simulink model "SingleTrackCANoe"  (R2021b)
settings: Solver=ode1  StartTime=0  StopTime=2  FixedStep=1.0000000000000000e-003  RelTol=1e-3
InitFcn:
  | sampleTime = str2double(get_param(bdroot, 'FixedStep'));
undefined symbols (not defined in the file or in its folder): AccPedalPos, BrakePedalPos, BrakeSwitch, DiscIntNeverNeededParam, DYNA4, EngSpd, IgnitionSwitch, InitialGear, InitialSpeed, IntendedEngTrq, LeftIndicator, MainBrakePress, MaxGear, MDL, MinGear, RefAcc, RefLane, RefLatPos, RefPath, RefPathCurv, RefSpd, RefSpdPreview, RefSpdRetrospect, RightIndicator, SteeringWheelAng, SteeringWheelTrq, UserDefinedRefValue, vm_const
libraries: UtilitiesLibrary x62, simulink x18, WheelSystemModules x14, LongitudinalControllerModules x13, LateralControllerModules x7, AnimationBusselectorModules x5, EnvironmentModules x5, BasicEngineControlModules x5, MiscellaneousControlModules x5, Animation3Modules x4, AuxiliariesModules x4, ReducedTireModules x4
(part 13 of 34)

== system SingleTrackCANoe/SimulationModel/Vehicle/Engine/EnginePhysics ==
  fromEngineControlUnit : Inport
  fromCTRL : Inport  Port=2
  fromEnvironment : Inport  Port=3
  fromChassis : Inport  Port=4
  fromDrivetrain : Inport  Port=5
  fromElectricalSystem : Inport  Port=6
  ConsumptionCalculation : EngineLookupTableModules/ConsumptionCalculation  FuelConsumptionLimStandEu=50  FuelConsumptionLimitCutoffUS=50
  DynaComponentInfo : Subsystem  Tag=DynaComponentInfo
      mask init:
      | data= get_param(gcb, 'UserData');
      settings: OpenFcn=DYNA4.ModelHandling.Component.ShowEditComponentInformationDialog(gcb);
      mask Display: disp(['Type = ', data.type, '\nGroup = ', data.group, '\nName = ', data.name ])
  EnginePhysicsOutput : Subsystem  Tag=TESIS DYNAware Interface Block  mask{NeedsUpdate=off, SignalInfo=|}
      mask SignalInfo=|
      | {
      |   "Version": "4.6",
      |   "MuxedOutputBusName": "EnginePhysics",
      |   "MuxedInputBusName": "input",
      |   "MuxedInputSelected": false,
      |   "MuxedOutputSelected": true,
      |   "SignalData": [
      |     {
      |       "initialValue": "0.0",
      |       "name": "Mechanics",
      |       "comment": "",
      |       "minString": "",
      |       "maxString": "",
      |       "width": -1,
      |       "dataType": 0,
      |       "signalType": 1,
      |       "createSignal": false,
      |       "outputName": "Mechanics",
      |       "generateSignalAccessBlock": false,
      |       "accessId": "$(parentId).$(blockName).$(outputName)"
      |     },
      |     {
      |       "initialValue": "0.0",
      |       "name": "ValidityStatus",
      |       "comment": "",
      |       "minString": "",
      |       "maxString": "",
      |       "width": -1,
      |       "dataType": 0,
      |       "signalType": 1,
      |       "createSignal": false,
      |       "outputName": "ValidityStatus",
      |       "generateSignalAccessBlock": false,
      |       "accessId": "$(parentId).$(blockName).$(outputName)"
      |     },
      |     {
      |       "initialValue": "0.0",
      |       "name": "FuelSystem",
      |       "comment": "",
      |       "minString": "",
      |       "maxString": "",
      |       "width": -1,
      |       "dataType": 0,
      |       "signalType": 1,
      |       "createSignal": false,
      |       "outputName": "FuelSystem",
      |       "generateSignalAccessBlock": false,
      |       "accessId": "$(parentId).$(blockName).$(outputName)"
      |     }
      |   ]
      | }
      mask prompts: NeedsUpdate "Specify, if subsystem content needs to be updated"; SignalInfo "Signal Info (json)"
      mask help: DYNA4 Interface Block Version 4.6
      mask init:
      | blockName = get_param(gcbh, 'Name');
      | parentId = DYNA4.ModelHandling.AccessID.getFromHierarchy(gcbh);
      | TD.InterfaceBlock.ModelCallbacks.GenerateContent(gcb);
      settings: DeleteFcn=TD.InterfaceBlock.ModelCallbacks.CloseGUI( gcbh );  NameChangeFcn=TD.InterfaceBlock.ModelCallbacks.BlockRenamedHandler(gcbh);  OpenFcn=TD.InterfaceBlock.ModelCallbacks.OpenGUI( gcbh );  CloseFcn=TD.InterfaceBlock.ModelCallbacks.CloseGUI( gcbh );
      mask Display:
      | image('InterfaceBlock.png','center');
      | port_label('input',1, 'Mechanics');
      | port_label('input',2, 'ValidityStatus');
      | port_label('input',3, 'FuelSystem');
      | port_label('output',1, 'EnginePhysics');
  FuelSystemOutput : Subsystem  Tag=TESIS DYNAware Interface Block  mask{NeedsUpdate=off, SignalInfo=|}
      mask SignalInfo=|
      | {
      |   "Version": "4.6",
      |   "MuxedOutputBusName": "FuelSystem",
      |   "MuxedInputBusName": "input",
      |   "MuxedInputSelected": false,
      |   "MuxedOutputSelected": true,
      |   "SignalData": [
      |     {
      |       "initialValue": "0.0",
      |       "name": "FuelMassFlow[kg/s]",
      |       "comment": "",
      |       "minString": "",
      |       "maxString": "",
      |       "width": 1,
      |       "dataType": 0,
      |       "signalType": 0,
      |       "createSignal": false,
      |       "outputName": "FuelMassFlow[kg/s]",
      |       "generateSignalAccessBlock": false,
      |       "accessId": "$(parentId).$(blockName).$(outputName)"
      |     },
      |     {
      |       "initialValue": "0.0",
      |       "name": "FuelMass[kg]",
      |       "comment": "",
      |       "minString": "",
      |       "maxString": "",
      |       "width": 1,
      |       "dataType": 0,
      |       "signalType": 0,
      |       "createSignal": false,
      |       "outputName": "FuelMass[kg]",
      |       "generateSignalAccessBlock": false,
      |       "accessId": "$(parentId).$(blockName).$(outputName)"
      |     },
      |     {
      |       "initialValue": "0.0",
      |       "name": "CurrFuelConsumEu[l/100km]",
      |       "comment": "",
      |       "minString": "",
      |       "maxString": "",
      |       "width": 1,
      |       "dataType": 0,
      |       "signalType": 0,
      |       "createSignal": false,
      |       "outputName": "CurrFuelConsumEu[l/100km]",
      |       "generateSignalAccessBlock": false,
      |       "accessId": "$(parentId).$(blockName).$(outputName)"
      |     },
      |     {
      |       "initialValue": "0.0",
      |       "name": "CurrFuelConsumUs[mpg]",
      |       "comment": "",
      |       "minString": "",
      |       "maxString": "",
      |       "width": 1,
      |       "dataType": 0,
      |       "signalType": 0,
      |       "createSignal": false,
      |       "outputName": "CurrFuelConsumUs[mpg]",
      |       "generateSignalAccessBlock": false,
      |       "accessId": "$(parentId).$(blockName).$(outputName)"
      |     },
      |     {
      |       "initialValue": "0.0",
      |       "name": "AvgFuelConsumEu[l/100km]",
      |       "comment": "",
      |       "minString": "",
      |       "maxString": "",
      |       "width": 1,
      |       "dataType": 0,
      |       "signalType": 0,
      |       "createSignal": false,
      |       "outputName": "AvgFuelConsumEu[l/100km]",
      |       "generateSignalAccessBlock": false,
      |       "accessId": "$(parentId).$(blockName).$(outputName)"
      |     },
      |     {
      |       "initialValue": "0.0",
      |       "name": "AvgFuelConsumUs[mpg]",
      |       "comment": "",
      |       "minString": "",
      |       "maxString": "",
      |       "width": 1,
      |       "dataType": 0,
      |       "signalType": 0,
      |       "createSignal": false,
      |       "outputName": "AvgFuelConsumUs[mpg]",
      |       "generateSignalAccessBlock": false,
      |       "accessId": "$(parentId).$(blockName).$(outputName)"
      |     },
      |     {
      |       "initialValue": "0.0",
      |       "name": "Efficiency[-]",
      |       "comment": "",
      |       "minString": "",
      |       "maxString": "",
      |       "width": 1,
      |       "dataType": 0,
      |       "signalType": 0,
      |       "createSignal": false,
      |       "outputName": "Efficiency[-]",
      |       "generateSignalAccessBlock": false,
      |       "accessId": "$(parentId).$(blockName).$(outputName)"
      |     },
      |     {
      |       "initialValue": "0.0",
      |       "name": "FuelDensity[kg/m**3]",
      |       "comment": "",
      |       "minString": "",
      |       "maxString": "",
      |       "width": 1,
      |       "dataType": 0,
      |       "signalType": 0,
      |       "createSignal": false,
      |       "outputName": "FuelDensity[kg/m**3]",
      |       "generateSignalAccessBlock": false,
      |       "accessId": "$(parentId).$(blockName).$(outputName)"
      |     }
      |   ]
      | }
      mask prompts: NeedsUpdate "Specify, if subsystem content needs to be updated"; SignalInfo "Signal Info (json)"
      mask help: DYNA4 Interface Block Version 4.6
      mask init:
      | blockName = get_param(gcbh, 'Name');
      | parentId = DYNA4.ModelHandling.AccessID.getFromHierarchy(gcbh);
      | TD.InterfaceBlock.ModelCallbacks.GenerateContent(gcb);
      settings: DeleteFcn=TD.InterfaceBlock.ModelCallbacks.CloseGUI( gcbh );  NameChangeFcn=TD.InterfaceBlock.ModelCallbacks.BlockRenamedHandler(gcbh);  OpenFcn=TD.InterfaceBlock.ModelCallbacks.OpenGUI( gcbh );  CloseFcn=TD.InterfaceBlock.ModelCallbacks.CloseGUI( gcbh );
      mask Display:
      | image('InterfaceBlock.png','center');
      | port_label('input',1, 'FuelMassFlow[kg/s]');
      | port_label('input',2, 'FuelMass[kg]');
      | port_label('input',3, 'CurrFuelConsumEu[l/100km]');
      | port_label('input',4, 'CurrFuelConsumUs[mpg]');
      | port_label('input',5, 'AvgFuelConsumEu[l/100km]');
      | port_label('input',6, 'AvgFuelConsumUs[mpg]');
      | port_label('input',7, 'Efficiency[-]');
      | port_label('input',8, 'FuelDensity[kg/m**3]');
      | port_label('output',1, 'FuelSystem');
  InputFromChassis : Subsystem  Tag=TESIS DYNAware Interface Block  mask{NeedsUpdate=off, SignalInfo=|}
      mask SignalInfo=|
      | {
      |   "Version": "4.6",
      |   "MuxedOutputBusName": "VEHICLE",
      |   "MuxedInputBusName": "fromChassis",
      |   "MuxedInputSelected": true,
      |   "MuxedOutputSelected": false,
      |   "SignalData": {
      |     "initialValue": "0.0",
      |     "name": "VehicleBody.AbsVel[m/s]",
      |     "comment": "",
      |     "minString": "",
      |     "maxString": "",
      |     "width": -1,
      |     "dataType": 0,
      |     "signalType": 0,
      |     "createSignal": false,
      |     "outputName": "AbsVel[m/s]",
      |     "generateSignalAccessBlock": false,
      |     "accessId": "$(parentId).$(blockName).$(outputName)"
      |   }
      | }
      mask prompts: NeedsUpdate "Specify, if subsystem content needs to be updated"; SignalInfo "Signal Info (json)"
      mask help: DYNA4 Interface Block Version 4.6
      mask init:
      | blockName = get_param(gcbh, 'Name');
      | parentId = DYNA4.ModelHandling.AccessID.getFromHierarchy(gcbh);
      | TD.InterfaceBlock.ModelCallbacks.GenerateContent(gcb);
      settings: DeleteFcn=TD.InterfaceBlock.ModelCallbacks.CloseGUI( gcbh );  NameChangeFcn=TD.InterfaceBlock.ModelCallbacks.BlockRenamedHandler(gcbh);  OpenFcn=TD.InterfaceBlock.ModelCallbacks.OpenGUI( gcbh );  CloseFcn=TD.InterfaceBlock.ModelCallbacks.CloseGUI( gcbh );
      mask Display:
      | image('InterfaceBlock.png','center');
      | port_label('input',1, 'fromChassis');
      | port_label('output',1, 'AbsVel[m/s]');
  InputFromDrivetrain : Subsystem  Tag=TESIS DYNAware Interface Block  mask{NeedsUpdate=off, SignalInfo=|}
      mask SignalInfo=|
      | {
      |   "Version": "4.6",
      |   "MuxedOutputBusName": "VEHICLE",
      |   "MuxedInputBusName": "fromDrivetrain",
      |   "MuxedInputSelected": true,
      |   "MuxedOutputSelected": false,
      |   "SignalData": {
      |     "initialValue": "0.0",
      |     "name": "DrivetrainPhysics.EngSpd[rad/s]",
      |     "comment": "",
      |     "minString": "",
      |     "maxString": "",
      |     "width": -1,
      |     "dataType": 0,
      |     "signalType": 0,
      |     "createSignal": false,
      |     "outputName": "EngSpd[rad/s]",
      |     "generateSignalAccessBlock": false,
      |     "accessId": "$(parentId).$(blockName).$(outputName)"
      |   }
      | }
      mask prompts: NeedsUpdate "Specify, if subsystem content needs to be updated"; SignalInfo "Signal Info (json)"
      mask help: DYNA4 Interface Block Version 4.6
      mask init:
      | blockName = get_param(gcbh, 'Name');
      | parentId = DYNA4.ModelHandling.AccessID.getFromHierarchy(gcbh);
      | TD.InterfaceBlock.ModelCallbacks.GenerateContent(gcb);
      settings: DeleteFcn=TD.InterfaceBlock.ModelCallbacks.CloseGUI( gcbh );  NameChangeFcn=TD.InterfaceBlock.ModelCallbacks.BlockRenamedHandler(gcbh);  OpenFcn=TD.InterfaceBlock.ModelCallbacks.OpenGUI( gcbh );  CloseFcn=TD.InterfaceBlock.ModelCallbacks.CloseGUI( gcbh );
      mask Display:
      | image('InterfaceBlock.png','center');
      | port_label('input',1, 'fromDrivetrain');
      | port_label('output',1, 'EngSpd[rad/s]');
  InputFromEngineControlUnit : Subsystem  Tag=TESIS DYNAware Interface Block  mask{NeedsUpdate=off, SignalInfo=|}
      mask SignalInfo=|
      | {
      |   "Version": "4.6",
      |   "MuxedOutputBusName": "VEHICLE",
      |   "MuxedInputBusName": "fromEngineControlUnit",
      |   "MuxedInputSelected": true,
      |   "MuxedOutputSelected": false,
      |   "SignalData": [
      |     {
      |       "initialValue": "0.0",
      |       "name": "EngLoadSignal[0_1]",
      |       "comment": "",
      |       "minString": "",
      |       "maxString": "",
      |       "width": -1,
      |       "dataType": 0,
      |       "signalType": 0,
      |       "createSignal": false,
      |       "outputName": "EngLoadSignal[0_1]",
      |       "generateSignalAccessBlock": false,
      |       "accessId": "$(parentId).$(blockName).$(outputName)"
      |     },
      |     {
      |       "initialValue": "0.0",
      |       "name": "EngFuelCutoff[0;1]",
      |       "comment": "",
      |       "minString": "",
      |       "maxString": "",
      |       "width": -1,
      |       "dataType": 0,
      |       "signalType": 0,
      |       "createSignal": false,
      |       "outputName": "EngFuelCutoff[0;1]",
      |       "generateSignalAccessBlock": false,
      |       "accessId": "$(parentId).$(blockName).$(outputName)"
      |     },
      |     {
      |       "initialValue": "0.0",
      |       "name": "UpperEngTrqSwitch[0;2]",
      |       "comment": "",
      |       "minString": "",
      |       "maxString": "",
      |       "width": -1,
      |       "dataType": 0,
      |       "signalType": 0,
      |       "createSignal": false,
      |       "outputName": "UpperEngTrqSwitch[0;2]",
      |       "generateSignalAccessBlock": false,
      |       "accessId": "$(parentId).$(blockName).$(outputName)"
      |     },
      |     {
      |       "initialValue": "0.0",
      |       "name": "UpperEngTrqLimit[Nm]",
      |       "comment": "",
      |       "minString": "",
      |       "maxString": "",
      |       "width": -1,
      |       "dataType": 0,
      |       "signalType": 0,
      |       "createSignal": false,
      |       "outputName": "UpperEngTrqLimit[Nm]",
      |       "generateSignalAccessBlock": false,
      |       "accessId": "$(parentId).$(blockName).$(outputName)"
      |     },
      |     {
      |       "initialValue": "0.0",
      |       "name": "LowerEngTrqSwitch[0;2]",
      |       "comment": "",
      |       "minString": "",
      |       "maxString": "",
      |       "width": -1,
      |       "dataType": 0,
      |       "signalType": 0,
      |       "createSignal": false,
      |       "outputName": "LowerEngTrqSwitch[0;2]",
      |       "generateSignalAccessBlock": false,
      |       "accessId": "$(parentId).$(blockName).$(outputName)"
      |     },
      |     {
      |       "initialValue": "0.0",
      |       "name": "LowerEngTrqLimit[Nm]",
      |       "comment": "",
      |       "minString": "",
      |       "maxString": "",
      |       "width": -1,
      |       "dataType": 0,
      |       "signalType": 0,
      |       "createSignal": false,
      |       "outputName": "LowerEngTrqLimit[Nm]",
      |       "generateSignalAccessBlock": false,
      |       "accessId": "$(parentId).$(blockName).$(outputName)"
      |     }
      |   ]
      | }
      mask prompts: NeedsUpdate "Specify, if subsystem content needs to be updated"; SignalInfo "Signal Info (json)"
      mask help: DYNA4 Interface Block Version 4.6
      mask init:
      | blockName = get_param(gcbh, 'Name');
      | parentId = DYNA4.ModelHandling.AccessID.getFromHierarchy(gcbh);
      | TD.InterfaceBlock.ModelCallbacks.GenerateContent(gcb);
      settings: DeleteFcn=TD.InterfaceBlock.ModelCallbacks.CloseGUI( gcbh );  NameChangeFcn=TD.InterfaceBlock.ModelCallbacks.BlockRenamedHandler(gcbh);  OpenFcn=TD.InterfaceBlock.ModelCallbacks.OpenGUI( gcbh );  CloseFcn=TD.InterfaceBlock.ModelCallbacks.CloseGUI( gcbh );
      mask Display:
      | image('InterfaceBlock.png','center');
      | port_label('input',1, 'fromEngineControlUnit');
      | port_label('output',1, 'EngLoadSignal[0_1]');
      | port_label('output',2, 'EngFuelCutoff[0;1]');
      | port_label('output',3, 'UpperEngTrqSwitch[0;2]');
      | port_label('output',4, 'UpperEngTrqLimit[Nm]');
      | port_label('output',5, 'LowerEngTrqSwitch[0;2]');
      | port_label('output',6, 'LowerEngTrqLimit[Nm]');
  MechanicsOutput : Subsystem  Tag=TESIS DYNAware Interface Block  mask{NeedsUpdate=off, SignalInfo=|}
      mask SignalInfo=|
      | {
      |   "Version": "4.6",
      |   "MuxedOutputBusName": "Mechanics",
      |   "MuxedInputBusName": "input",
      |   "MuxedInputSelected": false,
      |   "MuxedOutputSelected": true,
      |   "SignalData": [
      |     {
      |       "initialValue": "0.0",
      |       "name": "EngTrq[Nm]",
      |       "comment": "",
      |       "minString": "",
      |       "maxString": "",
      |       "width": 1,
      |       "dataType": 0,
      |       "signalType": 0,
      |       "createSignal": false,
      |       "outputName": "EngTrq[Nm]",
      |       "generateSignalAccessBlock": false,
      |       "accessId": "$(parentId).$(blockName).$(outputName)"
      |     },
      |     {
      |       "initialValue": "0.0",
      |       "name": "MeanEngTrq[Nm]",
      |       "comment": "",
      |       "minString": "",
      |       "maxString": "",
      |       "width": 1,
      |       "dataType": 0,
      |       "signalType": 0,
      |       "createSignal": false,
      |       "outputName": "MeanEngTrq[Nm]",
      |       "generateSignalAccessBlock": false,
      |       "accessId": "$(parentId).$(blockName).$(outputName)"
      |     },
      |     {
      |       "initialValue": "0.0",
      |       "name": "IndicatedTrq[Nm]",
      |       "comment": "",
      |       "minString": "",
      |       "maxString": "",
      |       "width": 1,
      |       "dataType": 0,
      |       "signalType": 0,
      |       "createSignal": false,
      |       "outputName": "IndicatedTrq[Nm]",
      |       "generateSignalAccessBlock": false,
      |       "accessId": "$(parentId).$(blockName).$(outputName)"
      |     },
      |     {
      |       "initialValue": "0.0",
      |       "name": "MeanIndicatedTrq[Nm]",
      |       "comment": "",
      |       "minString": "",
      |       "maxString": "",
      |       "width": 1,
      |       "dataType": 0,
      |       "signalType": 0,
      |       "createSignal": false,
      |       "outputName": "MeanIndicatedTrq[Nm]",
      |       "generateSignalAccessBlock": false,
      |       "accessId": "$(parentId).$(blockName).$(outputName)"
      |     },
      |     {
      |       "initialValue": "0.0",
      |       "name": "MeanEngFrictionTrq[Nm]",
      |       "comment": "",
      |       "minString": "",
      |       "maxString": "",
      |       "width": 1,
      |       "dataType": 0,
      |       "signalType": 0,
      |       "createSignal": false,
      |       "outputName": "MeanEngFrictionTrq[Nm]",
      |       "generateSignalAccessBlock": false,
      |       "accessId": "$(parentId).$(blockName).$(outputName)"
      |     },
      |     {
      |       "initialValue": "0.0",
      |       "name": "MeanEngDragTrq[Nm]",
      |       "comment": "",
      |       "minString": "",
      |       "maxString": "",
      |       "width": 1,
      |       "dataType": 0,
      |       "signalType": 0,
      |       "createSignal": false,
      |       "outputName": "MeanEngDragTrq[Nm]",
      |       "generateSignalAccessBlock": false,
      |       "accessId": "$(parentId).$(blockName).$(outputName)"
      |     },
      |     {
      |       "initialValue": "0.0",
      |       "name": "UnrestrictedEngTrq[Nm]",
      |       "comment": "",
      |       "minString": "",
      |       "maxString": "",
      |       "width": 1,
      |       "dataType": 0,
      |       "signalType": 0,
      |       "createSignal": false,
      |       "outputName": "UnrestrictedEngTrq[Nm]",
      |       "generateSignalAccessBlock": false,
      |       "accessId": "$(parentId).$(blockName).$(outputName)"
      |     },
      |     {
      |       "initialValue": "0.0",
      |       "name": "EngPow[W]",
      |       "comment": "",
      |       "minString": "",
      |       "maxString": "",
      |       "width": 1,
      |       "dataType": 0,
      |       "signalType": 0,
      |       "createSignal": false,
      |       "outputName": "EngPow[W]",
      |       "generateSignalAccessBlock": false,
      |       "accessId": "$(parentId).$(blockName).$(outputName)"
      |     },
      |     {
      |       "initialValue": "0.0",
      |       "name": "EngInrt[kg*m**2]",
      |       "comment": "",
      |       "minString": "",
      |       "maxString": "",
      |       "width": 1,
      |       "dataType": 0,
      |       "signalType": 0,
      |       "createSignal": false,
      |       "outputName": "EngInrt[kg*m**2]",
      |       "generateSignalAccessBlock": false,
      |       "accessId": "$(parentId).$(blockName).$(outputName)"
      |     },
      |     {
      |       "initialValue": "0.0",
      |       "name": "MeanEngMaxTrq[Nm]",
      |       "comment": "",
      |       "minString": "",
      |       "maxString": "",
      |       "width": 1,
      |       "dataType": 0,
      |       "signalType": 0,
      |       "createSignal": false,
      |       "outputName": "MeanEngMaxTrq[Nm]",
      |       "generateSignalAccessBlock": false,
      |       "accessId": "$(parentId).$(blockName).$(outputName)"
      |     },
      |     {
      |       "initialValue": "0.0",
      |       "name": "ThirtyPercentAccPedalEngTrq[Nm]",
      |       "comment": "",
      |       "minString": "",
      |       "maxString": "",
      |       "width": 1,
      |       "dataType": 0,
      |       "signalType": 0,
      |       "createSignal": false,
      |       "outputName": "ThirtyPercentAccPedalEngTrq[Nm]",
      |       "generateSignalAccessBlock": false,
      |       "accessId": "$(parentId).$(blockName).$(outputName)"
      |     },
      |     {
      |       "initialValue": "0.0",
      |       "name": "",
      |       "comment": "",
      |       "minString": "",
      |       "maxString": "",
      |       "width": 1,
      |       "dataType": 0,
      |       "signalType": 0,
      |       "createSignal": true,
      |       "outputName": "CrankAng[rad]",
      |       "generateSignalAccessBlock": false,
      |       "accessId": "$(parentId).$(blockName).$(outputName)"
      |     },
      |     {
      |       "initialValue": "0.0",
      |       "name": "",
      |       "comment": "",
      |       "minString": "",
      |       "maxString": "",
      |       "width": 1,
      |       "dataType": 0,
      |       "signalType": 0,
      |       "createSignal": true,
      |       "outputName": "DerivativeOfEngTrq_wrt_CrankAng[Nm/rad]",
      |       "generateSignalAccessBlock": false,
      |       "accessId": "$(parentId).$(blockName).$(outputName)"
      |     },
      |     {
      |       "initialValue": "0.0",
      |       "name": "",
      |       "comment": "",
      |       "minString": "",
      |       "maxString": "",
      |       "width": 1,
      |       "dataType": 0,
      |       "signalType": 0,
      |       "createSignal": true,
      |       "outputName": "DerivativeOfEngTrq_wrt_EngSpd[Nm/(rad/s)]",
      |       "generateSignalAccessBlock": false,
      |       "accessId": "$(parentId).$(blockName).$(outputName)"
      |     }
      |   ]
      | }
      mask prompts: NeedsUpdate "Specify, if subsystem content needs to be updated"; SignalInfo "Signal Info (json)"
      mask help: DYNA4 Interface Block Version 4.6
      mask init:
      | blockName = get_param(gcbh, 'Name');
      | parentId = DYNA4.ModelHandling.AccessID.getFromHierarchy(gcbh);
      | TD.InterfaceBlock.ModelCallbacks.GenerateContent(gcb);
      settings: DeleteFcn=TD.InterfaceBlock.ModelCallbacks.CloseGUI( gcbh );  NameChangeFcn=TD.InterfaceBlock.ModelCallbacks.BlockRenamedHandler(gcbh);  OpenFcn=TD.InterfaceBlock.ModelCallbacks.OpenGUI( gcbh );  CloseFcn=TD.InterfaceBlock.ModelCallbacks.CloseGUI( gcbh );
      settings: AttributesFormatString=|
      | CrankAng[rad] = 0.0
      | DerivativeOfEngTrq_wrt_CrankAng[Nm/rad] = 0.0
      | DerivativeOfEngTrq_wrt_EngSpd[Nm/(rad/s)] = 0.0
      mask Display:
      | image('InterfaceBlock.png','center');
      | port_label('input',1, 'EngTrq[Nm]');
      | port_label('input',2, 'MeanEngTrq[Nm]');
      | port_label('input',3, 'IndicatedTrq[Nm]');
      | port_label('input',4, 'MeanIndicatedTrq[Nm]');
      | port_label('input',5, 'MeanEngFrictionTrq[Nm]');
      | port_label('input',6, 'MeanEngDragTrq[Nm]');
      | port_label('input',7, 'UnrestrictedEngTrq[Nm]');
      | port_label('input',8, 'EngPow[W]');
      | port_label('input',9, 'EngInrt[kg*m**2]');
      | port_label('input',10, 'MeanEngMaxTrq[Nm]');
      | port_label('input',11, 'ThirtyPercentAccPedalEngTrq[Nm]');
      | port_label('output',1, 'Mechanics');
  Memory{1..3,5} (4 alike) : Memory  InheritSampleTime=on
  Mux : Mux
  TabledEngineTorque : EngineLookupTableModules/TabledEngineTorque  Tag=vedynaEngineMask  local_comp_inst=1  system_comp_inst=1  DATA_NODE=MDL.Vehicle.Engine.EnginePhysics.TabledEngineTorque  sample_time=-1
  TabledFuelConsumption : EngineLookupTableModules/TabledFuelConsumption  Tag=vedynaTabledConsumptionMask  DATA_NODE=MDL.Vehicle.Engine.EnginePhysics.TabledFuelConsumption  FuelDensity=MDL.Vehicle.Engine.EnginePhysics.TabledFuelConsumption.FuelDensity  NetCalorificValue=MDL.Vehicle.Engine.EnginePhysics.TabledFuelConsumption.NetCalorificValue  EngConsMap=MDL.Vehicle.Engine.EnginePhysics.TabledFuelConsumption.EngConsumptionMap
  Terminator : Terminator
  Terminator1 : Terminator
  Terminator2 : Terminator
  ValidityStatus : Subsystem  Tag=TESIS DYNAware Interface Block  mask{NeedsUpdate=off, SignalInfo=|}
      mask SignalInfo=|
      | {
      |   "Version": "4.6",
      |   "MuxedOutputBusName": "ValidityStatus",
      |   "MuxedInputBusName": "input",
      |   "MuxedInputSelected": false,
      |   "MuxedOutputSelected": true,
      |   "SignalData": {
      |     "initialValue": "0.0",
      |     "name": "ValidRangeExceededFlags[-]",
      |     "comment": "",
      |     "minString": "",
      |     "maxString": "",
      |     "width": 1,
      |     "dataType": 0,
      |     "signalType": 0,
      |     "createSignal": false,
      |     "outputName": "ValidRangeExceededFlags[-]",
      |     "generateSignalAccessBlock": false,
      |     "accessId": "$(parentId).$(blockName).$(outputName)"
      |   }
      | }
      mask prompts: NeedsUpdate "Specify, if subsystem content needs to be updated"; SignalInfo "Signal Info (json)"
      mask help: DYNA4 Interface Block Version 4.6
      mask init:
      | blockName = get_param(gcbh, 'Name');
      | parentId = DYNA4.ModelHandling.AccessID.getFromHierarchy(gcbh);
      | TD.InterfaceBlock.ModelCallbacks.GenerateContent(gcb);
      settings: DeleteFcn=TD.InterfaceBlock.ModelCallbacks.CloseGUI( gcbh );  NameChangeFcn=TD.InterfaceBlock.ModelCallbacks.BlockRenamedHandler(gcbh);  OpenFcn=TD.InterfaceBlock.ModelCallbacks.OpenGUI( gcbh );  CloseFcn=TD.InterfaceBlock.ModelCallbacks.CloseGUI( gcbh );
      mask Display:
      | image('InterfaceBlock.png','center');
      | port_label('input',1, 'ValidRangeExceededFlags[-]');
      | port_label('output',1, 'ValidityStatus');
  EnginePhysics : Outport  VectorParamsAs1DForOutWhenUnconnected=off
  wires:
  TabledFuelConsumption/2 -> FuelSystemOutput/7(Efficiency[-]___UNIQUE_1)
  ConsumptionCalculation/5 -> FuelSystemOutput/6(AvgFuelConsumUs[mpg]___UNIQUE_1)
  ConsumptionCalculation/4 -> FuelSystemOutput/5(AvgFuelConsumEu[l/100km]___UNIQUE_1)
  ConsumptionCalculation/3 -> FuelSystemOutput/4(CurrFuelConsumUs[mpg]___UNIQUE_1)
  ConsumptionCalculation/2 -> FuelSystemOutput/3(CurrFuelConsumEu[l/100km]___UNIQUE_1)
  MechanicsOutput/1(Mechanics___UNIQUE_1) -> EnginePhysicsOutput/1(Mechanics___UNIQUE_1)
  Memory3/1 -> MechanicsOutput/11(ThirtyPercentAccPedalEngTrq[Nm]___UNIQUE_1)
  Memory2/1 -> MechanicsOutput/10(MeanEngMaxTrq[Nm]___UNIQUE_1)
  Memory1/1 -> MechanicsOutput/7(UnrestrictedEngTrq[Nm]___UNIQUE_1)
  Memory5/1 -> MechanicsOutput/5(MeanEngFrictionTrq[Nm]___UNIQUE_1), MechanicsOutput/6(MeanEngDragTrq[Nm]___UNIQUE_1)
  TabledEngineTorque/2 -> MechanicsOutput/4(MeanIndicatedTrq[Nm]___UNIQUE_1), MechanicsOutput/3(IndicatedTrq[Nm]___UNIQUE_1)
  TabledEngineTorque/8 -> Memory2/1
  TabledEngineTorque/3 -> Memory5/1
  TabledEngineTorque/6 -> MechanicsOutput/9(EngInrt[kg*m**2]___UNIQUE_1)
  ValidityStatus/1(ValidityStatus___UNIQUE_1) -> EnginePhysicsOutput/2(ValidityStatus___UNIQUE_1)
  TabledEngineTorque/7 -> ValidityStatus/1(ValidRangeExceededFlags[-]___UNIQUE_1)
  InputFromEngineControlUnit/2(EngFuelCutoff[0;1]___UNIQUE_1) -> TabledFuelConsumption/4
  TabledEngineTorque/1 -> TabledFuelConsumption/3, MechanicsOutput/1(EngTrq[Nm]___UNIQUE_1), MechanicsOutput/2(MeanEngTrq[Nm]___UNIQUE_1)
  fromElectricalSystem/1 -> Terminator2/1
  EnginePhysicsOutput/1(EnginePhysics___UNIQUE_1) -> EnginePhysics/1
  fromChassis/1 -> InputFromChassis/1(fromChassis)
  fromDrivetrain/1 -> InputFromDrivetrain/1(fromDrivetrain)
  fromEngineControlUnit/1 -> InputFromEngineControlUnit/1(fromEngineControlUnit)
  InputFromDrivetrain/1(EngSpd[rad/s]) -> TabledEngineTorque/1, TabledFuelConsumption/2
  InputFromEngineControlUnit/3(UpperEngTrqSwitch[0;2]___UNIQUE_1) -> Mux/1
  InputFromEngineControlUnit/4(UpperEngTrqLimit[Nm]___UNIQUE_1) -> Mux/2
  InputFromEngineControlUnit/6(LowerEngTrqLimit[Nm]___UNIQUE_1) -> Mux/4
  InputFromEngineControlUnit/5(LowerEngTrqSwitch[0;2]___UNIQUE_1) -> Mux/3
  Mux/1 -> TabledEngineTorque/3
  FuelSystemOutput/1(FuelSystem___UNIQUE_1) -> EnginePhysicsOutput/3(FuelSystem___UNIQUE_1)
  ConsumptionCalculation/1 -> FuelSystemOutput/2(FuelMass[kg]___UNIQUE_1)
  fromEnvironment/1 -> Terminator/1
  TabledFuelConsumption/1 -> ConsumptionCalculation/1, FuelSystemOutput/1(FuelMassFlow[kg/s]___UNIQUE_1)
  TabledFuelConsumption/3 -> ConsumptionCalculation/2, FuelSystemOutput/8(FuelDensity[kg/m**3]___UNIQUE_1)
  TabledEngineTorque/5 -> MechanicsOutput/8(EngPow[W]___UNIQUE_1), TabledFuelConsumption/1
  TabledEngineTorque/4 -> Memory1/1
  InputFromEngineControlUnit/1(EngLoadSignal[0_1]___UNIQUE_1) -> TabledEngineTorque/2
  InputFromChassis/1(AbsVel[m/s]___UNIQUE_1) -> ConsumptionCalculation/3
  fromCTRL/1 -> Terminator1/1
  TabledEngineTorque/9 -> Memory3/1

== system SingleTrackCANoe/SimulationModel/Vehicle/VehicleRoadInfo/AdditionalRoadElevationAndRoadSlopes ==
  YawAng[rad] : Inport
  FrontLeftAddRoadElev[m] : Inport  Port=2
  FrontRightAddRoadElev[m] : Inport  Port=3
  AddLongRoadSlopeIn[-] : Inport  Port=4
  AddLatRoadSlopeIn[-] : Inport  Port=5
  LocalRoadSysSwitch[0;1] : Inport  Port=6
  Convert2VehSys : Subsystem
  Demux3 : Demux  Outputs=2
  Mux : Mux  Inputs=2
  Sum2 : Sum
  Switch : Switch  Criteria=u2 > Threshold  Threshold=0.5
  mean : Gain  Gain=0.5
  FrontAdditionalRoadElev[m] : Outport  VectorParamsAs1DForOutWhenUnconnected=off
  AddLongRoadSlope[-] : Outport  Port=2  VectorParamsAs1DForOutWhenUnconnected=off
  AddLatRoadSlope[-] : Outport  Port=3  VectorParamsAs1DForOutWhenUnconnected=off
  wires:
  YawAng[rad]/1 -> Convert2VehSys/1(YawAng[rad])
  Convert2VehSys/1(RoadSlopes(VehSys)) -> Switch/1
  Demux3/2 -> AddLatRoadSlope[-]/1
  Sum2/1 -> mean/1
  Demux3/1 -> AddLongRoadSlope[-]/1
  Mux/1 -> Switch/3, Convert2VehSys/2(RoadSlopes(WorldSys))
  FrontLeftAddRoadElev[m]/1 -> Sum2/1
  Switch/1 -> Demux3/1
  AddLongRoadSlopeIn[-]/1 -> Mux/1
  FrontRightAddRoadElev[m]/1 -> Sum2/2
  AddLatRoadSlopeIn[-]/1 -> Mux/2
  LocalRoadSysSwitch[0;1]/1 -> Switch/2
  mean/1 -> FrontAdditionalRoadElev[m]/1

== system SingleTrackCANoe/SimulationModel/Vehicle/VehicleRoadInfo/DynaComponentInfo ==

== system SingleTrackCANoe/SimulationModel/Vehicle/VehicleRoadInfo/InputFromCTRL ==
  fromCTRL : Inport
  TDBusSelector : BusSelector  OutputSignals=CTRL.AdditionalRoadElevation.FrontLeftAddRoadElev[m],CTRL.AdditionalRoadElevation.FrontRightAddRoadElev[m],CTRL.AdditionalRoadElevation.AddLongRoadSlope[-],CTRL.AdditionalRoadElevation.AddLatRoadSlope[-],CTRL.AdditionalRoadElevation.LocalRoadSysSwitch[0;1]
  __TDD__AddLatRoadSlope[-] : Demux  Outputs=[1]
  __TDD__AddLongRoadSlope[-] : Demux  Outputs=[1]
  __TDD__FrontLeftAddRoadElev[m] : Demux  Outputs=[1]
  __TDD__FrontRightAddRoadElev[m] : Demux  Outputs=[1]
  __TDD__LocalRoadSysSwitch[0;1] : Demux  Outputs=[1]
  FrontLeftAddRoadElev[m]___UNIQUE_1 : Outport  Description=|  PortDimensions=[1]  VectorParamsAs1DForOutWhenUnconnected=off
      | <name>CTRL.AdditionalRoadElevation.FrontLeftAddRoadElev[m]</name>
      | <comment></comment>
  FrontRightAddRoadElev[m]___UNIQUE_1 : Outport  Description=|  Port=2  PortDimensions=[1]  VectorParamsAs1DForOutWhenUnconnected=off
      | <name>CTRL.AdditionalRoadElevation.FrontRightAddRoadElev[m]</name>
      | <comment></comment>
  AddLongRoadSlope[-]___UNIQUE_1 : Outport  Description=|  Port=3  PortDimensions=[1]  VectorParamsAs1DForOutWhenUnconnected=off
      | <name>CTRL.AdditionalRoadElevation.AddLongRoadSlope[-]</name>
      | <comment></comment>
  AddLatRoadSlope[-]___UNIQUE_1 : Outport  Description=|  Port=4  PortDimensions=[1]  VectorParamsAs1DForOutWhenUnconnected=off
      | <name>CTRL.AdditionalRoadElevation.AddLatRoadSlope[-]</name>
      | <comment></comment>
  LocalRoadSysSwitch[0;1]___UNIQUE_1 : Outport  Description=|  Port=5  PortDimensions=[1]  VectorParamsAs1DForOutWhenUnconnected=off
      | <name>CTRL.AdditionalRoadElevation.LocalRoadSysSwitch[0;1]</name>
      | <comment></comment>
  wires:
  __TDD__LocalRoadSysSwitch[0;1]/1 -> LocalRoadSysSwitch[0;1]___UNIQUE_1/1  "LocalRoadSysSwitch[0;1]"
  __TDD__AddLatRoadSlope[-]/1 -> AddLatRoadSlope[-]___UNIQUE_1/1  "AddLatRoadSlope[-]"
  __TDD__AddLongRoadSlope[-]/1 -> AddLongRoadSlope[-]___UNIQUE_1/1  "AddLongRoadSlope[-]"
  __TDD__FrontRightAddRoadElev[m]/1 -> FrontRightAddRoadElev[m]___UNIQUE_1/1  "FrontRightAddRoadElev[m]"
  __TDD__FrontLeftAddRoadElev[m]/1 -> FrontLeftAddRoadElev[m]___UNIQUE_1/1  "FrontLeftAddRoadElev[m]"
  TDBusSelector/5 -> __TDD__LocalRoadSysSwitch[0;1]/1  "<LocalRoadSysSwitch[0;1]>"
  TDBusSelector/4 -> __TDD__AddLatRoadSlope[-]/1  "<AddLatRoadSlope[-]>"
  TDBusSelector/3 -> __TDD__AddLongRoadSlope[-]/1  "<AddLongRoadSlope[-]>"
  TDBusSelector/2 -> __TDD__FrontRightAddRoadElev[m]/1  "<FrontRightAddRoadElev[m]>"
  TDBusSelector/1 -> __TDD__FrontLeftAddRoadElev[m]/1  "<FrontLeftAddRoadElev[m]>"
  fromCTRL/1 -> TDBusSelector/1

== system SingleTrackCANoe/SimulationModel/Vehicle/VehicleRoadInfo/InputFromChassis ==
  fromChassis : Inport
  TDBusSelector : BusSelector  OutputSignals=VehicleBody.Pos(WorldSys)[m],VehicleBody.YawAng[rad]
  __TDD__Pos(WorldSys)[m] : Demux  Outputs=[3]
  __TDD__YawAng[rad] : Demux  Outputs=[1]
  Pos(WorldSys)[m]___UNIQUE_1 : Outport  Description=|  PortDimensions=[3]  VectorParamsAs1DForOutWhenUnconnected=off
      | <name>VehicleBody.Pos(WorldSys)[m]</name>
      | <comment></comment>
  YawAng[rad]___UNIQUE_1 : Outport  Description=|  Port=2  PortDimensions=[1]  VectorParamsAs1DForOutWhenUnconnected=off
      | <name>VehicleBody.YawAng[rad]</name>
      | <comment></comment>
  wires:
  __TDD__YawAng[rad]/1 -> YawAng[rad]___UNIQUE_1/1  "YawAng[rad]"
  __TDD__Pos(WorldSys)[m]/1 -> Pos(WorldSys)[m]___UNIQUE_1/1  "Pos(WorldSys)[m]"
  TDBusSelector/2 -> __TDD__YawAng[rad]/1  "<YawAng[rad]>"
  TDBusSelector/1 -> __TDD__Pos(WorldSys)[m]/1  "<Pos(WorldSys)[m]>"
  fromChassis/1 -> TDBusSelector/1

== system SingleTrackCANoe/SimulationModel/Vehicle/VehicleRoadInfo/VehicleRoadInfoOutput ==
  TrackID[-]___UNIQUE_1 : Inport  Description=|  PortDimensions=[1]
      | <name>TrackID[-]</name>
      | <comment></comment>
  LaneID[-]___UNIQUE_1 : Inport  Description=|  Port=2  PortDimensions=[1]
      | <name>LaneID[-]</name>
      | <comment></comment>
  RoadZ[m]___UNIQUE_1 : Inport  Description=|  Port=3  PortDimensions=[1]
      | <name>RoadZ[m]</name>
      | <comment></comment>
  RoadS[m]___UNIQUE_1 : Inport  Description=|  Port=4  PortDimensions=[1]
      | <name>RoadS[m]</name>
      | <comment></comment>
  RoadQ[m]___UNIQUE_1 : Inport  Description=|  Port=5  PortDimensions=[1]
      | <name>RoadQ[m]</name>
      | <comment></comment>
  RoadAngle[rad]___UNIQUE_1 : Inport  Description=|  Port=6  PortDimensions=[1]
      | <name>RoadAngle[rad]</name>
      | <comment></comment>
  RoadCurvature[1/m]___UNIQUE_1 : Inport  Description=|  Port=7  PortDimensions=[1]
      | <name>RoadCurvature[1/m]</name>
      | <comment></comment>
  LaneCurvature[1/m]___UNIQUE_1 : Inport  Description=|  Port=8  PortDimensions=[1]
      | <name>LaneCurvature[1/m]</name>
      | <comment></comment>
  RoadTangentXY[-]___UNIQUE_1 : Inport  Description=|  Port=9  PortDimensions=[2]
      | <name>RoadTangentXY[-]</name>
      | <comment></comment>
  RoadSlopeLong[-]___UNIQUE_1 : Inport  Description=|  Port=10  PortDimensions=[1]
      | <name>RoadSlopeLong[-]</name>
      | <comment></comment>
  RoadSlopeLat[-]___UNIQUE_1 : Inport  Description=|  Port=11  PortDimensions=[1]
      | <name>RoadSlopeLat[-]</name>
      | <comment></comment>
  RoadFriction[-]___UNIQUE_1 : Inport  Description=|  Port=12  PortDimensions=[1]
      | <name>RoadFriction[-]</name>
      | <comment></comment>
  RoadSurfaceType[-]___UNIQUE_1 : Inport  Description=|  Port=13  PortDimensions=[1]
      | <name>RoadSurfaceType[-]</name>
      | <comment></comment>
  RoadRoughness[-]___UNIQUE_1 : Inport  Description=|  Port=14  PortDimensions=[1]
      | <name>RoadRoughness[-]</name>
      | <comment></comment>
  RouteLength[m]___UNIQUE_1 : Inport  Description=|  Port=15  PortDimensions=[1]
      | <name>RouteLength[m]</name>
      | <comment></comment>
  RouteClosed[-]___UNIQUE_1 : Inport  Description=|  Port=16  PortDimensions=[1]
      | <name>RouteClosed[-]</name>
      | <comment></comment>
  __TDD__VehicleRoadInfo.LaneCurvature[1/m] : Demux  Outputs=[1]
  __TDD__VehicleRoadInfo.LaneID[-] : Demux  Outputs=[1]
  __TDD__VehicleRoadInfo.RoadAngle[rad] : Demux  Outputs=[1]
  __TDD__VehicleRoadInfo.RoadCurvature[1/m] : Demux  Outputs=[1]
  __TDD__VehicleRoadInfo.RoadFriction[-] : Demux  Outputs=[1]
  __TDD__VehicleRoadInfo.RoadQ[m] : Demux  Outputs=[1]
  __TDD__VehicleRoadInfo.RoadRoughness[-] : Demux  Outputs=[1]
  __TDD__VehicleRoadInfo.RoadS[m] : Demux  Outputs=[1]
  __TDD__VehicleRoadInfo.RoadSlopeLat[-] : Demux  Outputs=[1]
  __TDD__VehicleRoadInfo.RoadSlopeLong[-] : Demux  Outputs=[1]
  __TDD__VehicleRoadInfo.RoadSurfaceType[-] : Demux  Outputs=[1]
  __TDD__VehicleRoadInfo.RoadTangentXY[-] : Demux  Outputs=[2]
  __TDD__VehicleRoadInfo.RoadZ[m] : Demux  Outputs=[1]
  __TDD__VehicleRoadInfo.RouteClosed[-] : Demux  Outputs=[1]
  __TDD__VehicleRoadInfo.RouteLength[m] : Demux  Outputs=[1]
  __TDD__VehicleRoadInfo.TrackID[-] : Demux  Outputs=[1]
  __TDO__VehicleRoadInfo : BusCreator  Inputs=16
  VehicleRoadInfo___UNIQUE_1 : Outport  Description=|  PortDimensions=[17]  VectorParamsAs1DForOutWhenUnconnected=off
      | <name>TrackID[-]</name>
      | <comment></comment>
  wires:
  __TDO__VehicleRoadInfo/1 -> VehicleRoadInfo___UNIQUE_1/1  "VehicleRoadInfo"
  __TDD__VehicleRoadInfo.RouteClosed[-]/1 -> __TDO__VehicleRoadInfo/16  "RouteClosed[-]"
  RouteClosed[-]___UNIQUE_1/1 -> __TDD__VehicleRoadInfo.RouteClosed[-]/1
  __TDD__VehicleRoadInfo.RouteLength[m]/1 -> __TDO__VehicleRoadInfo/15  "RouteLength[m]"
  RouteLength[m]___UNIQUE_1/1 -> __TDD__VehicleRoadInfo.RouteLength[m]/1
  __TDD__VehicleRoadInfo.RoadRoughness[-]/1 -> __TDO__VehicleRoadInfo/14  "RoadRoughness[-]"
  RoadRoughness[-]___UNIQUE_1/1 -> __TDD__VehicleRoadInfo.RoadRoughness[-]/1
  __TDD__VehicleRoadInfo.RoadSurfaceType[-]/1 -> __TDO__VehicleRoadInfo/13  "RoadSurfaceType[-]"
  RoadSurfaceType[-]___UNIQUE_1/1 -> __TDD__VehicleRoadInfo.RoadSurfaceType[-]/1
  __TDD__VehicleRoadInfo.RoadFriction[-]/1 -> __TDO__VehicleRoadInfo/12  "RoadFriction[-]"
  RoadFriction[-]___UNIQUE_1/1 -> __TDD__VehicleRoadInfo.RoadFriction[-]/1
  __TDD__VehicleRoadInfo.RoadSlopeLat[-]/1 -> __TDO__VehicleRoadInfo/11  "RoadSlopeLat[-]"
  RoadSlopeLat[-]___UNIQUE_1/1 -> __TDD__VehicleRoadInfo.RoadSlopeLat[-]/1
  __TDD__VehicleRoadInfo.RoadSlopeLong[-]/1 -> __TDO__VehicleRoadInfo/10  "RoadSlopeLong[-]"
  RoadSlopeLong[-]___UNIQUE_1/1 -> __TDD__VehicleRoadInfo.RoadSlopeLong[-]/1
  __TDD__VehicleRoadInfo.RoadTangentXY[-]/1 -> __TDO__VehicleRoadInfo/9  "RoadTangentXY[-]"
  RoadTangentXY[-]___UNIQUE_1/1 -> __TDD__VehicleRoadInfo.RoadTangentXY[-]/1
  __TDD__VehicleRoadInfo.LaneCurvature[1/m]/1 -> __TDO__VehicleRoadInfo/8  "LaneCurvature[1/m]"
  LaneCurvature[1/m]___UNIQUE_1/1 -> __TDD__VehicleRoadInfo.LaneCurvature[1/m]/1
  __TDD__VehicleRoadInfo.RoadCurvature[1/m]/1 -> __TDO__VehicleRoadInfo/7  "RoadCurvature[1/m]"
  RoadCurvature[1/m]___UNIQUE_1/1 -> __TDD__VehicleRoadInfo.RoadCurvature[1/m]/1
  __TDD__VehicleRoadInfo.RoadAngle[rad]/1 -> __TDO__VehicleRoadInfo/6  "RoadAngle[rad]"
  RoadAngle[rad]___UNIQUE_1/1 -> __TDD__VehicleRoadInfo.RoadAngle[rad]/1
  __TDD__VehicleRoadInfo.RoadQ[m]/1 -> __TDO__VehicleRoadInfo/5  "RoadQ[m]"
  RoadQ[m]___UNIQUE_1/1 -> __TDD__VehicleRoadInfo.RoadQ[m]/1
  __TDD__VehicleRoadInfo.RoadS[m]/1 -> __TDO__VehicleRoadInfo/4  "RoadS[m]"
  RoadS[m]___UNIQUE_1/1 -> __TDD__VehicleRoadInfo.RoadS[m]/1
  __TDD__VehicleRoadInfo.RoadZ[m]/1 -> __TDO__VehicleRoadInfo/3  "RoadZ[m]"
  RoadZ[m]___UNIQUE_1/1 -> __TDD__VehicleRoadInfo.RoadZ[m]/1
  __TDD__VehicleRoadInfo.LaneID[-]/1 -> __TDO__VehicleRoadInfo/2  "LaneID[-]"
  LaneID[-]___UNIQUE_1/1 -> __TDD__VehicleRoadInfo.LaneID[-]/1
  __TDD__VehicleRoadInfo.TrackID[-]/1 -> __TDO__VehicleRoadInfo/1  "TrackID[-]"
  TrackID[-]___UNIQUE_1/1 -> __TDD__VehicleRoadInfo.TrackID[-]/1

== system SingleTrackCANoe/SimulationModel/Vehicle/WheelSystem/DynaComponentInfo ==
